simulink model "p2_phase_loop_cosim_verification"  (Simulink 6.4)
settings: Solver=ode1  SolverMode=SingleTasking  StartTime=0.0  StopTime=8e-2  RelTol=1e-3
undefined symbols (not defined in the file or in its folder): pipeline_prec
libraries: simulink x4, modelsimlib x1
settings Model: LastModifiedBy=Administrador

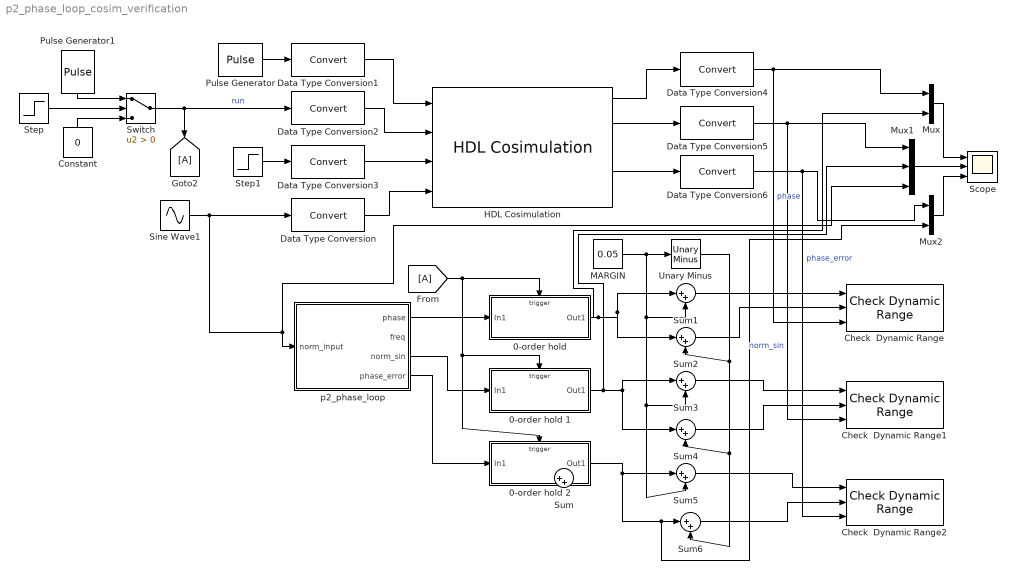
== system p2_phase_loop_cosim_verification ==
  0-order hold : Subsystem
  0-order hold 1 : Subsystem
  0-order hold 2 : Subsystem
  Check  Dynamic Range : simulink/Model Verification/Check  Dynamic Range  Description=min < sig < max  SystemSampleTime=-1  enabled=off  stopWhenAssertionFail=on  export=off  icon=graphic
  Check  Dynamic Range1 : simulink/Model Verification/Check  Dynamic Range  Description=min < sig < max  SystemSampleTime=-1  enabled=off  stopWhenAssertionFail=on  export=off  icon=graphic
  Check  Dynamic Range2 : simulink/Model Verification/Check  Dynamic Range  Description=min < sig < max  SystemSampleTime=-1  enabled=off  stopWhenAssertionFail=on  export=off  icon=graphic
  Constant : Constant  Orientation=up  Value=0  OutDataType=sfix(16)  ConRadixGroup=Use specified scaling  OutScaling=2^0  SampleTime=1e-7  FramePeriod=inf
  Data Type Conversion : DataTypeConversion  OutDataTypeMode=Specify via dialog  OutScaling=2^(-pipeline_prec)  RndMeth=Nearest  SaturateOnIntegerOverflow=on
  Data Type Conversion1 : DataTypeConversion  OutDataTypeMode=boolean  SampleTime=1e-7
  Data Type Conversion2 : DataTypeConversion  OutDataTypeMode=boolean
  Data Type Conversion3 : DataTypeConversion  OutDataTypeMode=boolean
  Data Type Conversion4 : DataTypeConversion
  Data Type Conversion5 : DataTypeConversion
  Data Type Conversion6 : DataTypeConversion
  HDL Cosimulation : modelsimlib/HDL Cosimulation  DialogController=modelsimddg.CoSim  DialogControllerArgs=DataTag0  PortPaths=/p2_phase_loop/clk;/p2_phase_loop/run;/p2_phase_loop/rst;/p2_phase_loop/input;/p2_phase_loop/phase;/p2_phase_loop/norm_sin;/p2_phase_loop/done;/p2_phase_loop/phase_det_i/phase_error;/p2_phase_loop/iir_1st_ord/o  PortModes=[1 1 1 1 2 2 2 2 2 ]  PortTimes=[1,1,1,1,1e-5,1e-5,1e-5,1e-5,1e-5]  PortSigns=[-1 -1 -1 -1 1 1 -1 1 1 ]  PortFracLengths=[0,0,0,0,pipeline_prec,pipeline_prec,0,pipeline_prec,pipeline_prec]  CommLocal=on  CommSharedMemory=off  CommPortNumber=4449  CommShowInfo=on  ClockModes=[]  ClockTimes=[]  TclPreSimCommand="echo \"Running Simulink Cosimulation block.\""  TclPostSimCommand="echo \"done\""  TimingMode=s  TimingScaleFactor=1  idxCellArray={'UNUSED_VAR'}
  MARGIN : Constant  Value=0.05  OutDataType=sfix(16)  ConRadixGroup=Use specified scaling  OutScaling=2^0  SampleTime=inf  FramePeriod=inf
  Mux : Mux  Inputs=2
  Mux1 : Mux  Inputs=3
  Mux2 : Mux  Inputs=2
  Pulse Generator : DiscretePulseGenerator  PulseType=Time based  Period=1/(1e6)  PulseWidth=50
  Pulse Generator1 : DiscretePulseGenerator  Orientation=down  PulseType=Time based  Period=0.1e-3  PulseWidth=2
  Scope : Scope  NumInputPorts=3
      settings: YMin=-4~-1.25~-5  YMax=7~1.25~5  MaxDataPoints=500000
  Sine Wave1 : Sin  Frequency=2*pi*50.05  Phase=1  SampleTime=1e-7
  Step : Step  Time=4*(1/1e6)  SampleTime=1e-7
  Step1 : Step  Time=6*(1/1e6)  Before=1  After=0  SampleTime=1e-7
  Sum{,1..6} (7 alike) : Sum  Inputs=|++
  Switch : Switch  Criteria=u2 > Threshold  RndMeth=Nearest  ZeroCross=off  SampleTime=1e-7
  Unary Minus : simulink/Math Operations/Unary Minus  DoSatur=off
  p2_phase_loop : Subsystem  TreatAsAtomicUnit=on
  wires:
  Data Type Conversion/1 -> HDL Cosimulation/4
  Sine Wave1/1 -> Data Type Conversion/1, p2_phase_loop/1(norm_input), Mux1/3
  Pulse Generator/1 -> Data Type Conversion1/1
  Data Type Conversion1/1 -> HDL Cosimulation/1
  Data Type Conversion2/1 -> HDL Cosimulation/2
  Step1/1 -> Data Type Conversion3/1
  Data Type Conversion3/1 -> HDL Cosimulation/3
  Constant/1 -> Switch/3
  Step/1 -> Switch/2
  Pulse Generator1/1 -> Switch/1
  HDL Cosimulation/1 -> Data Type Conversion4/1
  Data Type Conversion4/1 -> Check  Dynamic Range/3, Mux/1  "phase"
  Data Type Conversion5/1 -> Check  Dynamic Range1/3, Mux1/1  "norm_sin"
  Data Type Conversion6/1 -> Check  Dynamic Range2/3, Mux2/1  "phase_error"
  HDL Cosimulation/2 -> Data Type Conversion5/1
  p2_phase_loop/1(phase) -> 0-order hold/1(In1)
  p2_phase_loop/3(norm_sin) -> 0-order hold 1/1(In1)
  p2_phase_loop/4(phase_error) -> 0-order hold 2/1(In1)
  Switch/1 -> Data Type Conversion2/1, [A]  "run"
  [A] -> 0-order hold/Trigger, 0-order hold 1/Trigger, 0-order hold 2/Trigger
  HDL Cosimulation/4 -> Data Type Conversion6/1
  0-order hold/1(Out1) -> Sum1/1, Sum2/1, Mux/2
  Sum1/1 -> Check  Dynamic Range/1
  Sum2/1 -> Check  Dynamic Range/2
  0-order hold 1/1(Out1) -> Sum3/1, Sum4/1, Mux1/2
  Sum3/1 -> Check  Dynamic Range1/1
  Sum4/1 -> Check  Dynamic Range1/2
  0-order hold 2/1(Out1) -> Sum5/1, Sum6/1, Mux2/2
  Sum5/1 -> Check  Dynamic Range2/1
  Sum6/1 -> Check  Dynamic Range2/2
  MARGIN/1 -> Unary Minus/1, Sum1/2, Sum5/2, Sum3/2
  Unary Minus/1 -> Sum6/2, Sum4/2, Sum2/2
  Mux/1 -> Scope/1
  Mux1/1 -> Scope/2
  Mux2/1 -> Scope/3

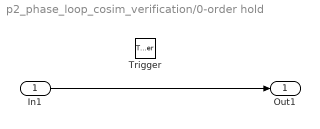
== system p2_phase_loop_cosim_verification/0-order hold ==
  In1 : Inport
  Trigger : TriggerPort  OutputDataType=double
  Out1 : Outport
  wires:
  In1/1 -> Out1/1

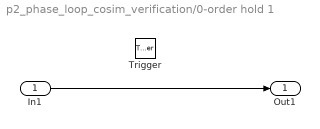
== system p2_phase_loop_cosim_verification/0-order hold 1 ==
  In1 : Inport
  Trigger : TriggerPort  OutputDataType=double
  Out1 : Outport
  wires:
  In1/1 -> Out1/1

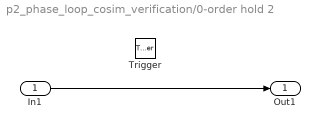
== system p2_phase_loop_cosim_verification/0-order hold 2 ==
  In1 : Inport
  Trigger : TriggerPort  OutputDataType=double
  Out1 : Outport
  wires:
  In1/1 -> Out1/1

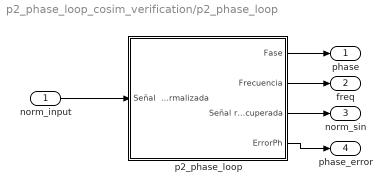
== system p2_phase_loop_cosim_verification/p2_phase_loop ==
  norm_input : Inport
  p2_phase_loop : Subsystem
  phase : Outport
  freq : Outport  Port=2
  norm_sin : Outport  Port=3
  phase_error : Outport  Port=4
  wires:
  norm_input/1 -> p2_phase_loop/1(Señal  normalizada)
  p2_phase_loop/1(Fase) -> phase/1
  p2_phase_loop/2(Frecuencia) -> freq/1
  p2_phase_loop/3(Señal recuperada) -> norm_sin/1
  p2_phase_loop/4(ErrorPh) -> phase_error/1

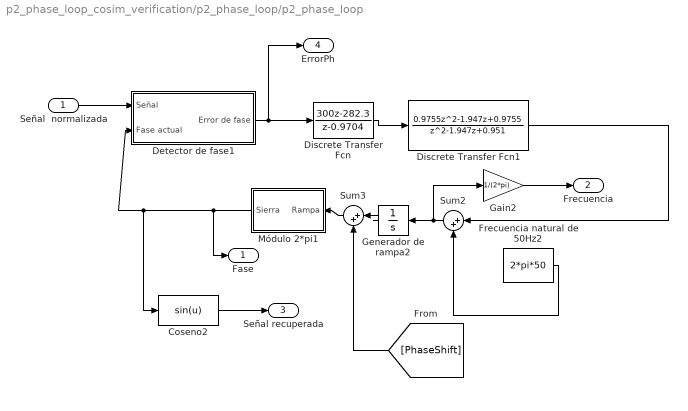
== system p2_phase_loop_cosim_verification/p2_phase_loop/p2_phase_loop ==
  Señal  normalizada : Inport
  Coseno2 : Fcn  Expr=sin(u)
  Detector de fase1 : Subsystem
  Discrete Transfer Fcn : DiscreteTransferFcn  Numerator=[300 -282.3]  Denominator=[1 -0.9704]  SampleTime=1e-4
  Discrete Transfer Fcn1 : DiscreteTransferFcn  Numerator=[0.9755 -1.947 0.9755]  Denominator=[1 -1.947 0.951]  SampleTime=1e-4
  Frecuencia natural de 50Hz2 : Constant  Value=2*pi*50  OutDataType=sfix(16)  ConRadixGroup=Use specified scaling  OutScaling=2^0  SampleTime=inf  FramePeriod=inf
  Gain2 : Gain  Gain=1/(2*pi)  SaturateOnIntegerOverflow=on
  Generador de rampa2 : Integrator  Orientation=left
  Módulo 2*pi1 : Subsystem  Orientation=left
  Sum2 : Sum  Orientation=left  Inputs=|++  SaturateOnIntegerOverflow=on
  Sum3 : Sum  Orientation=left  Inputs=|++  SaturateOnIntegerOverflow=on
  Fase : Outport
  Frecuencia : Outport  Port=2
  Señal recuperada : Outport  Port=3
  ErrorPh : Outport  Port=4
  wires:
  Módulo 2*pi1/1(Sierra) -> Fase/1, Detector de fase1/2(Fase actual), Coseno2/1
  Frecuencia natural de 50Hz2/1 -> Sum2/2
  Coseno2/1 -> Señal recuperada/1
  Sum2/1 -> Generador de rampa2/1, Gain2/1
  Señal  normalizada/1 -> Detector de fase1/1(Señal)
  Generador de rampa2/1 -> Sum3/1
  Sum3/1 -> Módulo 2*pi1/1(Rampa)
  [PhaseShift] -> Sum3/2
  Gain2/1 -> Frecuencia/1
  Discrete Transfer Fcn/1 -> Discrete Transfer Fcn1/1
  Detector de fase1/1(Error de fase) -> Discrete Transfer Fcn/1, ErrorPh/1
  Discrete Transfer Fcn1/1 -> Sum2/1

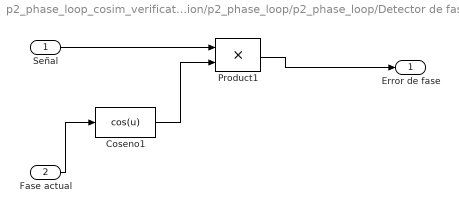
== system p2_phase_loop_cosim_verification/p2_phase_loop/p2_phase_loop/Detector de fase1 ==
  Señal : Inport
  Fase actual : Inport  Port=2
  Coseno1 : Fcn  Expr=cos(u)
  Product1 : Product  SaturateOnIntegerOverflow=on
  Error de fase : Outport
  wires:
  Señal/1 -> Product1/1
  Coseno1/1 -> Product1/2
  Fase actual/1 -> Coseno1/1
  Product1/1 -> Error de fase/1

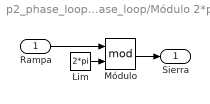
== system p2_phase_loop_cosim_verification/p2_phase_loop/p2_phase_loop/Módulo 2*pi1 ==
  Rampa : Inport
  " Módulo" : Math  Operator=mod  SaturateOnIntegerOverflow=on
  Lim : Constant  Value=2*pi  OutDataType=sfix(16)  ConRadixGroup=Use specified scaling  OutScaling=2^0  SampleTime=inf  FramePeriod=inf
  Sierra : Outport
  wires:
  Rampa/1 -> " Módulo"/1
  " Módulo"/1 -> Sierra/1
  Lim/1 -> " Módulo"/2
